simulink model "debug"  (R2022b)
settings: Solver=VariableStepAuto  StartTime=0.0  StopTime=20  RelTol=1e-3
settings Model: Creator=KarlO  LastModifiedBy=KarlO

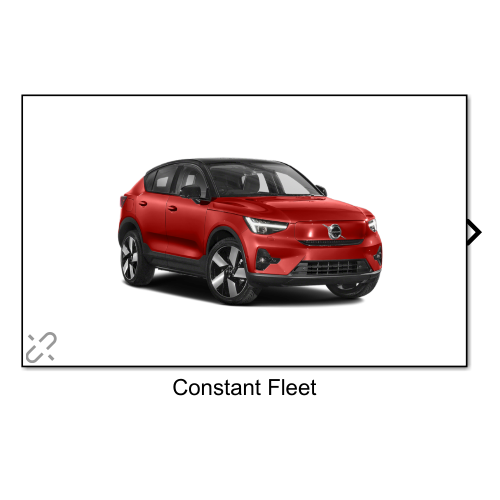
[thumbnail: Simulink's stored preview of the top-level diagram]
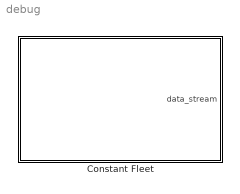
== system debug ==
  Constant Fleet : Subsystem  AncestorBlock=VACLib/Vehicle Components/Constant Fleet
      settings: LibrarySourceBlock=VACLib/Vehicle Components/Constant Fleet
      mask Display: image('C:\Users\KarlO\architectural-tradeoff-analysis\DCA-simulator\Volvo Architecture\VAC library\Images\VAC\cc9459c7a9e4acd4eb37509497aa20bf.png',[40,10,125,100]); % Use "Edit Image" on toolstrip to change.

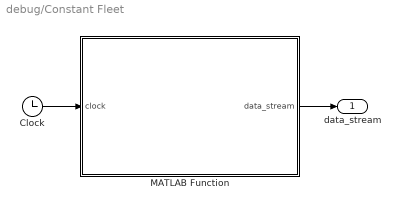
== system debug/Constant Fleet ==
  Clock : Clock
  MATLAB Function : MATLAB Function  TreatAsAtomicUnit=on
  data_stream : Outport
  wires:
  Clock/1 -> MATLAB Function/1(clock)
  MATLAB Function/1(data_stream) -> data_stream/1

== matlab function debug/Constant Fleet/MATLAB Function ==
  data: clock input; data_stream output
function data_stream  = fcn(clock)

persistent out;
persistent last_tick;
persistent data_to_send;

message_size = 1;
car_cache = 1;
fleet_size = 1000;
simulation_time = 10;

if isempty(out)
    out = 0;
    data_to_send = (message_size*fleet_size*simulation_time);
    last_tick = 0;
end

tick = clock;
passed_time = tick-last_tick;
last_tick = tick;

send_this_tick = (data_to_send/simulation_time)*passed_time;

to_send = floor(send_this_tick/(car_cache*message_size));

if tick >= simulation_time
    out = data_to_send;
else
    out = out + (to_send*car_cache*message_size);
end

data_stream = [out,(car_cache*message_size), fleet_size, simulation_time];
